simulink model "pendulum"  (R2023b)
settings: Solver=ode45  StartTime=0.0  StopTime=10  RelTol=1e-3
settings Model: Creator=yuanluochen  LastModifiedBy=yuanluochen

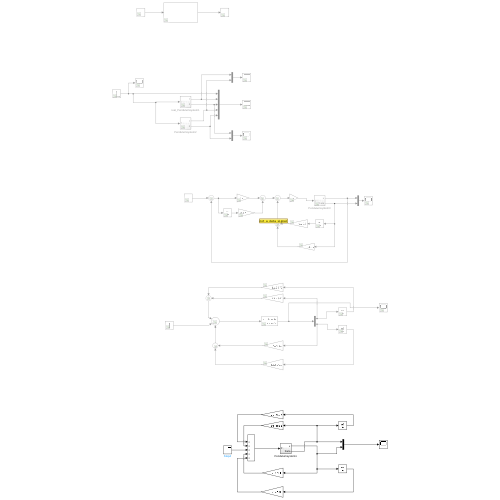
[thumbnail: Simulink's stored preview of the top-level diagram]
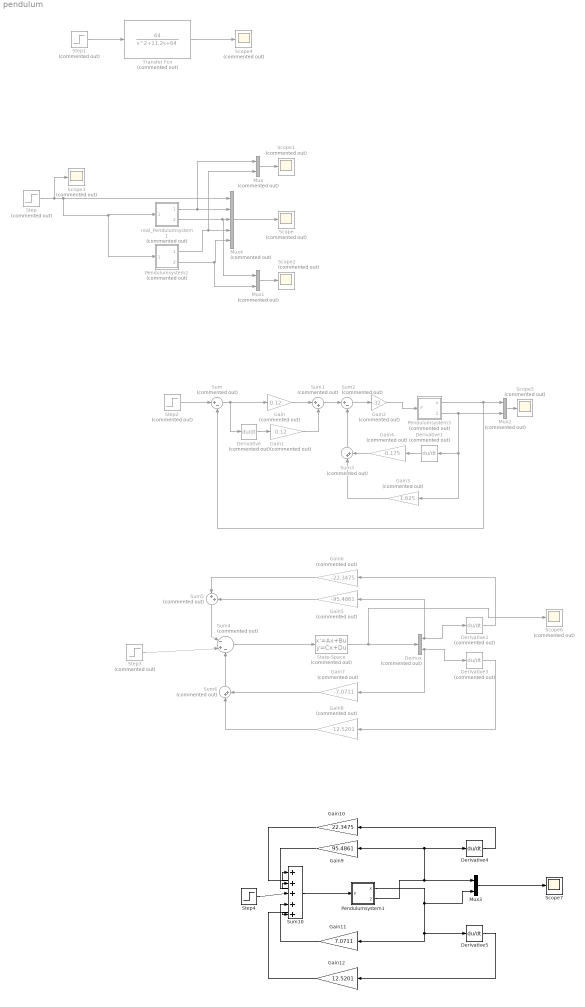
== system pendulum ==
  Demux : Demux  Commented=on  Outputs=2
  Derivative{,1..3} (4 alike) : Derivative  Commented=on
  Derivative4 : Derivative
  Derivative5 : Derivative
  Gain : Gain  Commented=on  Gain=0.12
  Gain1 : Gain  Commented=on  Gain=0.12
  Gain10 : Gain  Gain=22.3475
  Gain11 : Gain  Gain=7.0711
  Gain12 : Gain  Gain=12.5201
  Gain2 : Gain  Commented=on  Gain=-32
  Gain3 : Gain  Commented=on  Gain=1.625
  Gain4 : Gain  Commented=on  Gain=0.175
  Gain5 : Gain  Commented=on  Gain=-95.4861
  Gain6 : Gain  Commented=on  Gain=-22.3475
  Gain7 : Gain  Commented=on  Gain=-7.0711
  Gain8 : Gain  Commented=on  Gain=-12.5201
  Gain9 : Gain  Gain=95.4861
  Mux : Mux  Commented=on  Inputs=2
  Mux1 : Mux  Commented=on  Inputs=2
  Mux2 : Mux  Commented=on  Inputs=2
  Mux3 : Mux  Inputs=2
  Mux4 : Mux  Commented=on  Inputs=5
  Pendulumsystem1 : Subsystem
  Pendulumsystem2 : Subsystem  Commented=on
  Pendulumsystem3 : Subsystem  Commented=on
  Scope{,1..6} (7 alike) : Scope  Commented=on
  Scope7 : Scope
  State-Space : StateSpace  Commented=on  A=[0 1 0 0;40 0 0 0;0 0 0 1;-6 0 0 0]  B=[0;-2;0;0.8]  C=[1 0 0 0;0 0 1 0]  D=[0;0]  InitialCondition=0
  Step : Step  Commented=on  Time=0.1  Before=0.1  After=0  SampleTime=0
  Step1 : Step  Commented=on  Time=0  SampleTime=0
  Step2 : Step  Commented=on  Time=0  SampleTime=0
  Step3 : Step  Commented=on  Time=0  SampleTime=0
  Step4 : Step  Time=0  SampleTime=0
  Sum : Sum  Commented=on  Inputs=|+-
  Sum{1,3,5..6} (4 alike) : Sum  Commented=on  Inputs=|++
  Sum10 : Sum  Inputs=|+++++
  Sum2 : Sum  Commented=on  Inputs=|+-
  Sum4 : Sum  Commented=on  Inputs=|-+-
  Transfer Fcn : TransferFcn  Commented=on  Numerator=[64]  Denominator=[1 11.2 64]
  real_Pendulumsystem1 : Subsystem  Commented=on
  wires:
  Step/1 -> Scope3/1, Pendulumsystem2/1(In1), real_Pendulumsystem1/1(In1), Mux4/1
  Mux4/1 -> Scope/1
  real_Pendulumsystem1/1(Out1) -> Mux/1, Mux4/2
  real_Pendulumsystem1/2(Out2) -> Mux1/1, Mux4/3
  Pendulumsystem2/1(Out1) -> Mux/2, Mux4/4
  Pendulumsystem2/2(Out2) -> Mux1/2, Mux4/5
  Mux/1 -> Scope1/1
  Mux1/1 -> Scope2/1
  Step1/1 -> Transfer Fcn/1
  Transfer Fcn/1 -> Scope4/1
  Step2/1 -> Sum/1
  Sum/1 -> Derivative/1, Gain/1
  Derivative/1 -> Gain1/1
  Gain/1 -> Sum1/1
  Gain1/1 -> Sum1/2
  Sum1/1 -> Sum2/1
  Sum2/1 -> Gain2/1
  Gain2/1 -> Pendulumsystem3/1(F)
  Derivative1/1 -> Gain4/1
  Gain4/1 -> Sum3/2
  Sum3/1 -> Sum2/2
  Gain3/1 -> Sum3/1
  Mux2/1 -> Scope5/1
  Pendulumsystem3/1(x) -> Sum/2, Mux2/1
  Pendulumsystem3/2(theta) -> Gain3/1, Derivative1/1, Mux2/2
  Step3/1 -> Sum4/2
  Sum5/1 -> Sum4/1
  Sum6/1 -> Sum4/3
  Gain5/1 -> Sum5/2
  Gain6/1 -> Sum5/1
  Gain7/1 -> Sum6/2
  Gain8/1 -> Sum6/1
  Sum4/1 -> State-Space/1
  State-Space/1 -> Scope6/1, Demux/1
  Demux/1 -> Gain5/1, Derivative2/1
  Demux/2 -> Gain7/1, Derivative3/1
  Derivative2/1 -> Gain6/1
  Derivative3/1 -> Gain8/1
  Gain9/1 -> Sum10/2
  Pendulumsystem1/1(x) -> Gain11/1, Derivative5/1, Mux3/2
  Gain12/1 -> Sum10/5
  Gain11/1 -> Sum10/4
  Sum10/1 -> Pendulumsystem1/1(F)
  Pendulumsystem1/2(theta) -> Gain9/1, Derivative4/1, Mux3/1
  Step4/1 -> Sum10/3
  Derivative4/1 -> Gain10/1
  Gain10/1 -> Sum10/1
  Derivative5/1 -> Gain12/1
  Mux3/1 -> Scope7/1

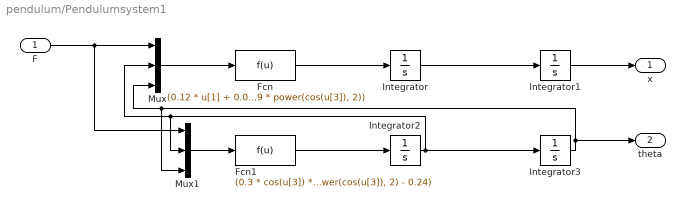
== system pendulum/Pendulumsystem1 ==
  F : Inport
  Fcn : Fcn  Expr=(0.12 * u[1] + 0.036 * sin(u[3]) * power(u[2], 2) - 0.9 * sin(u[3]) * cos(u[3]))/(0.24 - 0.09 * power(cos(u[3]), 2))
  Fcn1 : Fcn  Expr=(0.3 * cos(u[3]) * u[1] + 0.09 * sin(u[3]) * cos(u[3]) * power(u[2], 2) - 6 * sin(u[3]))/(0.09 * power(cos(u[3]), 2) - 0.24)
  Integrator{,1..3} (4 alike) : Integrator
  Mux : Mux  Inputs=3
  Mux1 : Mux  Inputs=3
  x : Outport
  theta : Outport  Port=2
  wires:
  Mux1/1 -> Fcn1/1
  Integrator2/1 -> Mux1/2, Mux/2, Integrator3/1
  Fcn/1 -> Integrator/1
  Mux/1 -> Fcn/1
  Integrator3/1 -> theta/1, Mux1/3, Mux/3
  Fcn1/1 -> Integrator2/1
  F/1 -> Mux/1, Mux1/1
  Integrator/1 -> Integrator1/1
  Integrator1/1 -> x/1

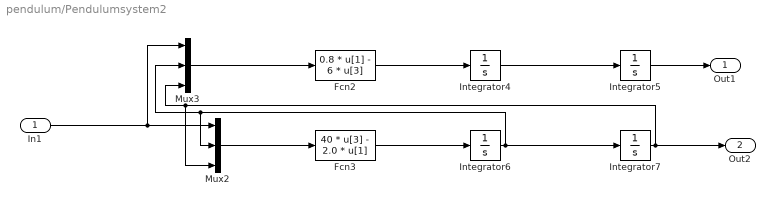
== system pendulum/Pendulumsystem2 ==
  In1 : Inport
  Fcn2 : Fcn  Expr=0.8 * u[1] - 6 * u[3]
  Fcn3 : Fcn  Expr=40 * u[3] - 2.0 * u[1]
  Integrator{4..7} (4 alike) : Integrator
  Mux2 : Mux  Inputs=3
  Mux3 : Mux  Inputs=3
  Out1 : Outport
  Out2 : Outport  Port=2
  wires:
  Mux2/1 -> Fcn3/1
  Fcn3/1 -> Integrator6/1
  Integrator6/1 -> Mux3/2, Mux2/2, Integrator7/1
  Integrator5/1 -> Out1/1
  Fcn2/1 -> Integrator4/1
  Integrator4/1 -> Integrator5/1
  Mux3/1 -> Fcn2/1
  In1/1 -> Mux2/1, Mux3/1
  Integrator7/1 -> Mux2/3, Mux3/3, Out2/1

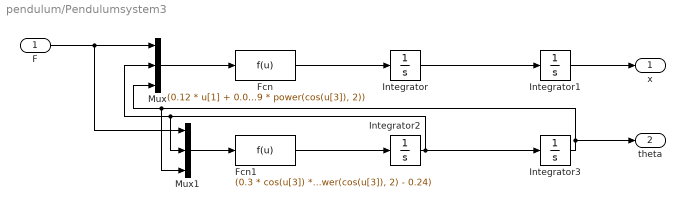
== system pendulum/Pendulumsystem3 ==
  F : Inport
  Fcn : Fcn  Expr=(0.12 * u[1] + 0.036 * sin(u[3]) * power(u[2], 2) - 0.9 * sin(u[3]) * cos(u[3]))/(0.24 - 0.09 * power(cos(u[3]), 2))
  Fcn1 : Fcn  Expr=(0.3 * cos(u[3]) * u[1] + 0.09 * sin(u[3]) * cos(u[3]) * power(u[2], 2) - 6 * sin(u[3]))/(0.09 * power(cos(u[3]), 2) - 0.24)
  Integrator{,1..3} (4 alike) : Integrator
  Mux : Mux  Inputs=3
  Mux1 : Mux  Inputs=3
  x : Outport
  theta : Outport  Port=2
  wires:
  Mux1/1 -> Fcn1/1
  Integrator2/1 -> Mux1/2, Mux/2, Integrator3/1
  Fcn/1 -> Integrator/1
  Mux/1 -> Fcn/1
  Integrator3/1 -> theta/1, Mux1/3, Mux/3
  Fcn1/1 -> Integrator2/1
  F/1 -> Mux/1, Mux1/1
  Integrator/1 -> Integrator1/1
  Integrator1/1 -> x/1

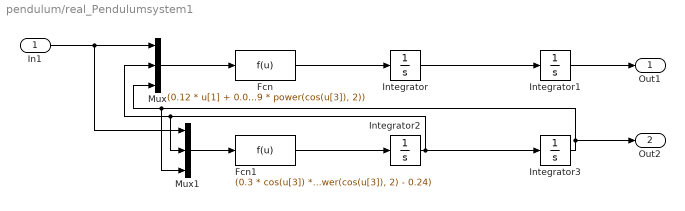
== system pendulum/real_Pendulumsystem1 ==
  In1 : Inport
  Fcn : Fcn  Expr=(0.12 * u[1] + 0.036 * sin(u[3]) * power(u[2], 2) - 0.9 * sin(u[3]) * cos(u[3]))/(0.24 - 0.09 * power(cos(u[3]), 2))
  Fcn1 : Fcn  Expr=(0.3 * cos(u[3]) * u[1] + 0.09 * sin(u[3]) * cos(u[3]) * power(u[2], 2) - 6 * sin(u[3]))/(0.09 * power(cos(u[3]), 2) - 0.24)
  Integrator{,1..3} (4 alike) : Integrator
  Mux : Mux  Inputs=3
  Mux1 : Mux  Inputs=3
  Out1 : Outport
  Out2 : Outport  Port=2
  wires:
  Mux1/1 -> Fcn1/1
  Integrator2/1 -> Mux1/2, Mux/2, Integrator3/1
  Fcn/1 -> Integrator/1
  Mux/1 -> Fcn/1
  Integrator3/1 -> Out2/1, Mux1/3, Mux/3
  Fcn1/1 -> Integrator2/1
  In1/1 -> Mux/1, Mux1/1
  Integrator/1 -> Integrator1/1
  Integrator1/1 -> Out1/1
